simulink model "PVArrayIVTestXaxisShade"  (R2023a)
settings: Solver=VariableStepAuto  StartTime=0.0  StopTime=10.0  RelTol=1e-3
undefined symbols (not defined in the file): Rl
libraries: spsSeriesRLCBranchLib x84, spsPVArrayLib x72, spsCurrentMeasurementLib x12, spsVariableResistorLib x12, spsVoltageMeasurementLib x12, SignalEditorBlockLib x1, sps_lib x1
settings Model: Creator=Akbar  LastModifiedBy=Akbar

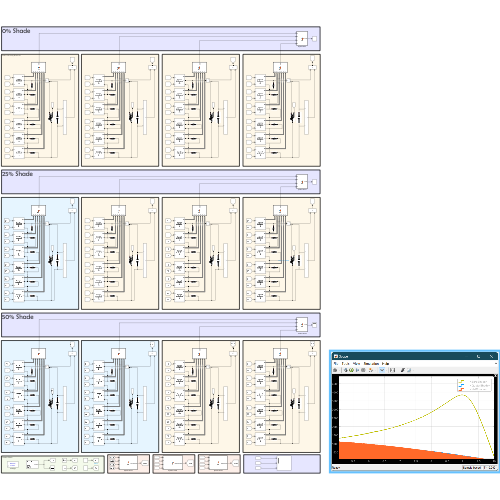
[thumbnail: Simulink's stored preview of the top-level diagram]
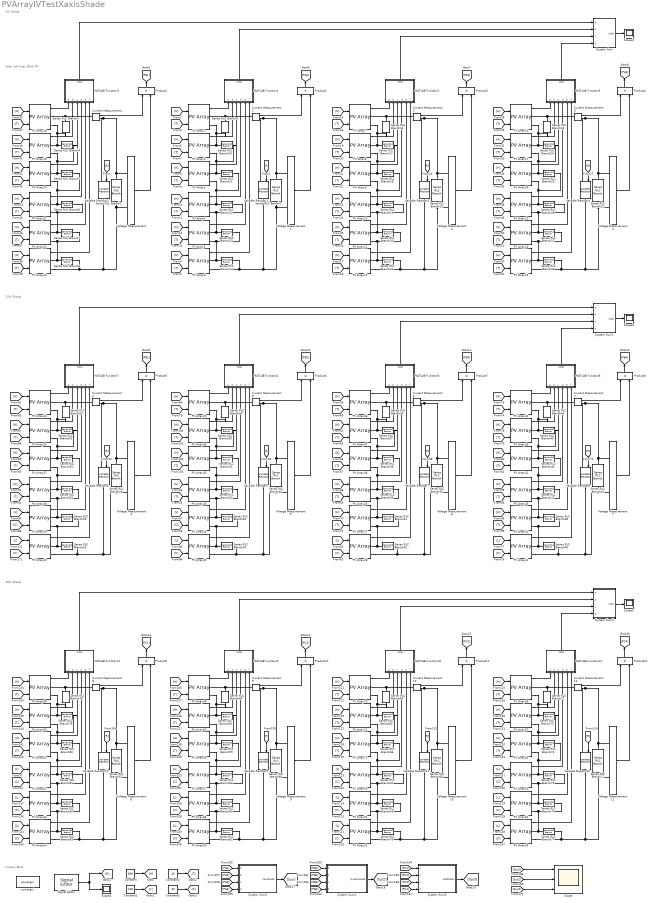
== system PVArrayIVTestXaxisShade ==
  note: Primary Block
  note: 0% Shade
  note: Solar Cell Array Block #1
  note: 25% Shade
  note: 50% Shade
  Constant : Constant  Value=800
  Constant1 : Constant  Value=100
  Constant2 : Constant  Value=45
  Constant3 : Constant  Value=30
  Current Measurement{,1..11} (12 alike) : spsCurrentMeasurementLib/Current Measurement  PhasorSimulation=off  OutputType=Complex  PSBequivalent=0
  MATLAB Function1 : MATLAB Function  TreatAsAtomicUnit=on
  MATLAB Function10 : MATLAB Function  TreatAsAtomicUnit=on
  MATLAB Function11 : MATLAB Function  TreatAsAtomicUnit=on
  MATLAB Function12 : MATLAB Function  TreatAsAtomicUnit=on
  MATLAB Function2 : MATLAB Function  TreatAsAtomicUnit=on
  MATLAB Function3 : MATLAB Function  TreatAsAtomicUnit=on
  MATLAB Function4 : MATLAB Function  TreatAsAtomicUnit=on
  MATLAB Function5 : MATLAB Function  TreatAsAtomicUnit=on
  MATLAB Function6 : MATLAB Function  TreatAsAtomicUnit=on
  MATLAB Function7 : MATLAB Function  TreatAsAtomicUnit=on
  MATLAB Function8 : MATLAB Function  TreatAsAtomicUnit=on
  MATLAB Function9 : MATLAB Function  TreatAsAtomicUnit=on
  PV Array{1..72} (72 alike) : spsPVArrayLib/PV Array  Npar=1  Nser=1  PlotType=array @ 1000 W/m2 & specified temperatures  S_vec="[ 1000  500  100 ]"  Temp_C_vec="[ 45 25  ]"  ModuleName=User-defined  PlotWhenSelected=off  Pm=213.15  Ncell=60  Voc=36.3  Isc=7.84  Vm=29  Im=7.35  beta_Voc_pc=-0.36099  alpha_Isc_pc=0.102  beta_Voc=-0.13104  alpha_Isc=0.0079968  IL=7.8654  I0=2.9273e-10  nI=0.98119  Rsh=313.0553  Rs=0.39381  RobustModel=off  RobustCellTemperature=313.3991  BAL=on  Tc=1e-6  Tfilter=5e-5
  Product{1..12} (12 alike) : Product
  Scope : Scope  NumInputPorts=3
  Scope{2..5} (4 alike) : Scope
  Series RLC Branch{1..2,15,22,29,35,40,43,57,63,68,71} (12 alike) : spsSeriesRLCBranchLib/Series RLC Branch  LConnTagsString=__new0  RConnTagsString=__new0  BranchType=C  Resistance=Rl  Inductance=1e-3  SetiL0=off  InitialCurrent=0  Capacitance=0.01  Setx0=off  InitialVoltage=150  Measurements=Branch voltage and current
  Series RLC Branch{3..14,16..21,23..28,30..34,36..39,41..42,44..56,58..62,64..67,69..70,72..84} (72 alike) : spsSeriesRLCBranchLib/Series RLC Branch  LConnTagsString=__new0  RConnTagsString=__new0  BranchType=C  Resistance=Rl  Inductance=1e-3  SetiL0=off  InitialCurrent=0  Capacitance=1e-2  Setx0=off  InitialVoltage=0  Measurements=Branch voltage and current
  Signal Editor : SignalEditorBlockLib/Signal Editor  FileName=C:\Users\Akbar\Cloud-Drive\School Work\L6 BEng EEE\Semester 1\EEE6016 Renewables\VR\Matlab\SlopeDown1000.mat  ActiveScenario=SlopeHalf  ActiveSignal=Posit  IsBus=off  OutputBusObjectStr=Bus: BusObject  SampleTime=0.0001  ZeroCross=off  OutputAfterFinalValue=Holding final value  Unit=inherit  PreserveSignalName=on  ApplySigPropsToAllScenarios=on
  System Sum : MATLAB Function  TreatAsAtomicUnit=on
  System Sum1 : MATLAB Function  TreatAsAtomicUnit=on
  System Sum2 : MATLAB Function  TreatAsAtomicUnit=on
  System Sum3 : MATLAB Function  TreatAsAtomicUnit=on
  System Sum4 : MATLAB Function  TreatAsAtomicUnit=on
  System Sum5 : MATLAB Function  TreatAsAtomicUnit=on
  Variable Resistor{1..12} (12 alike) : spsVariableResistorLib/Variable Resistor  Rabsmin=1e-3
      settings: LibrarySourceBlock=sps_lib/Passives/Variable Resistor
  Voltage Measurement{,1..11} (12 alike) : spsVoltageMeasurementLib/Voltage Measurement  PhasorSimulation=off  OutputType=Complex  PSBequivalent=0
  powergui : sps_lib/powergui  Priority=1  SimulationMode=Discrete  SampleTime=1e-6  frequency=60  Iterations=50  frequencyindice=0  Pbase=100e6  ErrMax=1e-4  UnitsV=kV  UnitsW=MW  buscounter=0  FunctionMessages=off  echomessages=off  EnableUseOfTLC=off  CurrentSourceSwitches=off  DisableSnubberDevices=off  DisableRonSwitches=off  DisableVfSwitches=off  DisplayEquations=off  AutomaticDiscreteSolvers=off  SolverType=Tustin/Backward Euler (TBE)  Interpol=off  ExternalGateDelay=off  methode=off  Ts=100  x0status=blocks  SPID=on  SwTol=0  HookPort=off  NonlinearTolerance=1e-4  nMaxIteration=100  ContinueOnMaxIteration=off  RestoreLinks=warning  ResistiveCurrentMeasurement=off  Frange=[0:2:500]  Ylog=off  Xlog=on  ShowGrid=off  save=off  variable=ZData  structure=0  ZoomFFT=off  StartTime=0.0  cycles=1  DisplayStyle=1  fundamental=60  FreqAxis=off  MaxFrequency=1000  frequencyindicesteady=1  RmsSteady=1  display=off
  wires:
  PV Array23/1 -> MATLAB Function3/6(f)
  [T] -> PV Array23/2
  [H] -> PV Array18/1
  PV Array19/1 -> MATLAB Function3/2(b)
  PV Array22/1 -> MATLAB Function3/5(e)
  [H] -> PV Array23/1
  [H] -> PV Array21/1
  PV Array20/1 -> MATLAB Function3/3(c)
  [H] -> PV Array22/1
  PV Array21/1 -> MATLAB Function3/4(d)
  [H] -> PV Array20/1
  PV Array18/1 -> MATLAB Function3/1(a)
  [T] -> PV Array19/2
  [H] -> PV Array19/1
  Constant1/1 -> [L]
  Constant/1 -> [H]
  Constant2/1 -> [T]
  Constant3/1 -> [C]
  [T] -> PV Array21/2
  [T] -> PV Array18/2
  [T] -> PV Array20/2
  [T] -> PV Array22/2
  Signal Editor/1 -> [R], Scope2/1
  System Sum/1(total) -> Scope3/1
  [R] -> Variable Resistor2/1
  [R] -> Variable Resistor1/1
  [H] -> PV Array3/1
  PV Array1/1 -> MATLAB Function1/1(a)
  [H] -> PV Array6/1
  [T] -> PV Array1/2
  PV Array4/1 -> MATLAB Function1/4(d)
  [T] -> PV Array4/2
  [T] -> PV Array3/2
  PV Array6/1 -> MATLAB Function1/6(f)
  [T] -> PV Array6/2
  [H] -> PV Array1/1
  [T] -> PV Array5/2
  [H] -> PV Array4/1
  [T] -> PV Array2/2
  PV Array3/1 -> MATLAB Function1/3(c)
  [H] -> PV Array2/1
  PV Array5/1 -> MATLAB Function1/5(e)
  PV Array2/1 -> MATLAB Function1/2(b)
  [H] -> PV Array5/1
  [R] -> Variable Resistor3/1
  [H] -> PV Array9/1
  PV Array7/1 -> MATLAB Function2/1(a)
  [H] -> PV Array12/1
  [T] -> PV Array7/2
  PV Array10/1 -> MATLAB Function2/4(d)
  [T] -> PV Array10/2
  [T] -> PV Array9/2
  PV Array12/1 -> MATLAB Function2/6(f)
  [T] -> PV Array12/2
  [H] -> PV Array7/1
  [T] -> PV Array11/2
  [H] -> PV Array10/1
  [T] -> PV Array8/2
  PV Array9/1 -> MATLAB Function2/3(c)
  [H] -> PV Array8/1
  PV Array11/1 -> MATLAB Function2/5(e)
  PV Array8/1 -> MATLAB Function2/2(b)
  [H] -> PV Array11/1
  [H] -> PV Array17/1
  PV Array24/1 -> MATLAB Function5/3(c)
  [T] -> PV Array17/2
  [H] -> PV Array13/1
  PV Array14/1 -> MATLAB Function5/5(e)
  PV Array15/1 -> MATLAB Function5/6(f)
  [H] -> PV Array15/1
  PV Array16/1 -> MATLAB Function5/1(a)
  [T] -> PV Array14/2
  PV Array13/1 -> MATLAB Function5/4(d)
  [H] -> PV Array16/1
  [R] -> Variable Resistor4/1
  [H] -> PV Array24/1
  [H] -> PV Array14/1
  [T] -> PV Array13/2
  PV Array17/1 -> MATLAB Function5/2(b)
  [T] -> PV Array15/2
  [T] -> PV Array24/2
  [T] -> PV Array16/2
  MATLAB Function5/1(total) -> System Sum/4(d)
  MATLAB Function2/1(total) -> System Sum/3(c)
  MATLAB Function1/1(total) -> System Sum/2(b)
  MATLAB Function3/1(total) -> System Sum/1(a)
  Voltage Measurement/1 -> Product1/2
  Current Measurement/1 -> Product1/1
  Voltage Measurement1/1 -> Product2/2
  Current Measurement1/1 -> Product2/1
  Voltage Measurement2/1 -> Product3/2
  Current Measurement2/1 -> Product3/1
  Voltage Measurement3/1 -> Product4/2
  Current Measurement3/1 -> Product4/1
  [H] -> PV Array29/1
  PV Array30/1 -> MATLAB Function8/5(e)
  PV Array36/1 -> MATLAB Function4/2(b)
  [H] -> PV Array25/1
  [T] -> PV Array43/2
  PV Array45/1 -> MATLAB Function4/6(f)
  PV Array43/1 -> MATLAB Function4/4(d)
  [T] -> PV Array36/2
  [R] -> Variable Resistor5/1
  [H] -> PV Array42/1
  [T] -> PV Array25/2
  PV Array25/1 -> MATLAB Function4/1(a)
  [T] -> PV Array42/2
  [H] -> PV Array43/1
  MATLAB Function6/1(total) -> System Sum1/3(c)
  Current Measurement6/1 -> Product7/1
  Current Measurement5/1 -> Product6/1
  PV Array31/1 -> MATLAB Function8/6(f)
  [T] -> PV Array30/2
  PV Array32/1 -> MATLAB Function8/1(a)
  [H] -> PV Array33/1
  MATLAB Function8/1(total) -> System Sum1/4(d)
  PV Array29/1 -> MATLAB Function8/4(d)
  [H] -> PV Array30/1
  [R] -> Variable Resistor8/1
  [H] -> PV Array41/1
  [T] -> PV Array29/2
  Current Measurement7/1 -> Product8/1
  Voltage Measurement7/1 -> Product8/2
  [T] -> PV Array32/2
  Voltage Measurement5/1 -> Product6/2
  Current Measurement4/1 -> Product5/1
  PV Array34/1 -> MATLAB Function7/1(a)
  PV Array37/1 -> MATLAB Function7/3(c)
  [H] -> PV Array36/1
  PV Array40/1 -> MATLAB Function7/6(f)
  Voltage Measurement6/1 -> Product7/2
  PV Array42/1 -> MATLAB Function4/3(c)
  PV Array39/1 -> MATLAB Function7/5(e)
  PV Array35/1 -> MATLAB Function7/2(b)
  MATLAB Function7/1(total) -> System Sum1/1(a)
  Voltage Measurement4/1 -> Product5/2
  [T] -> PV Array33/2
  [H] -> PV Array47/1
  PV Array48/1 -> MATLAB Function6/3(c)
  [T] -> PV Array47/2
  [H] -> PV Array26/1
  PV Array27/1 -> MATLAB Function6/5(e)
  [H] -> PV Array32/1
  PV Array28/1 -> MATLAB Function6/6(f)
  [T] -> PV Array27/2
  [H] -> PV Array46/1
  [H] -> PV Array48/1
  [R] -> Variable Resistor7/1
  [R] -> Variable Resistor6/1
  [H] -> PV Array27/1
  PV Array38/1 -> MATLAB Function7/4(d)
  PV Array47/1 -> MATLAB Function6/2(b)
  [T] -> PV Array48/2
  [T] -> PV Array46/2
  [T] -> PV Array26/2
  PV Array44/1 -> MATLAB Function4/5(e)
  PV Array26/1 -> MATLAB Function6/4(d)
  PV Array33/1 -> MATLAB Function8/2(b)
  PV Array41/1 -> MATLAB Function8/3(c)
  MATLAB Function4/1(total) -> System Sum1/2(b)
  PV Array46/1 -> MATLAB Function6/1(a)
  System Sum1/1(total) -> Scope4/1
  [T] -> PV Array41/2
  PV Array54/1 -> MATLAB Function12/5(e)
  PV Array60/1 -> MATLAB Function9/2(b)
  PV Array69/1 -> MATLAB Function9/6(f)
  PV Array67/1 -> MATLAB Function9/4(d)
  [R] -> Variable Resistor9/1
  PV Array49/1 -> MATLAB Function9/1(a)
  MATLAB Function10/1(total) -> System Sum2/3(c)
  Current Measurement10/1 -> Product11/1
  Current Measurement9/1 -> Product10/1
  PV Array55/1 -> MATLAB Function12/6(f)
  PV Array56/1 -> MATLAB Function12/1(a)
  [H] -> PV Array57/1
  MATLAB Function12/1(total) -> System Sum2/4(d)
  PV Array53/1 -> MATLAB Function12/4(d)
  [R] -> Variable Resistor12/1
  Current Measurement11/1 -> Product12/1
  Voltage Measurement11/1 -> Product12/2
  [T] -> PV Array56/2
  Voltage Measurement9/1 -> Product10/2
  Current Measurement8/1 -> Product9/1
  PV Array58/1 -> MATLAB Function11/1(a)
  PV Array61/1 -> MATLAB Function11/3(c)
  PV Array64/1 -> MATLAB Function11/6(f)
  Voltage Measurement10/1 -> Product11/2
  PV Array66/1 -> MATLAB Function9/3(c)
  PV Array63/1 -> MATLAB Function11/5(e)
  PV Array59/1 -> MATLAB Function11/2(b)
  MATLAB Function11/1(total) -> System Sum2/1(a)
  Voltage Measurement8/1 -> Product9/2
  [T] -> PV Array57/2
  [H] -> PV Array71/1
  PV Array72/1 -> MATLAB Function10/3(c)
  [T] -> PV Array71/2
  PV Array51/1 -> MATLAB Function10/5(e)
  [H] -> PV Array56/1
  PV Array52/1 -> MATLAB Function10/6(f)
  [H] -> PV Array70/1
  [R] -> Variable Resistor11/1
  [R] -> Variable Resistor10/1
  PV Array62/1 -> MATLAB Function11/4(d)
  PV Array71/1 -> MATLAB Function10/2(b)
  [T] -> PV Array70/2
  PV Array68/1 -> MATLAB Function9/5(e)
  PV Array50/1 -> MATLAB Function10/4(d)
  PV Array57/1 -> MATLAB Function12/2(b)
  PV Array65/1 -> MATLAB Function12/3(c)
  MATLAB Function9/1(total) -> System Sum2/2(b)
  PV Array70/1 -> MATLAB Function10/1(a)
  System Sum2/1(total) -> Scope5/1
  Product1/1 -> [PA1]
  Product2/1 -> [PA2]
  Product3/1 -> [PA3]
  Product4/1 -> [PA4]
  Product5/1 -> [PB1]
  Product6/1 -> [PB2]
  Product7/1 -> [PB3]
  Product8/1 -> [PB4]
  Product9/1 -> [PC1]
  Product10/1 -> [PC2]
  Product11/1 -> [PC3]
  Product12/1 -> [PC4]
  [PA1] -> System Sum3/1(a)
  [PA2] -> System Sum3/2(b)
  [PA3] -> System Sum3/3(c)
  [PA4] -> System Sum3/4(d)
  System Sum3/1(ZeroShade) -> [Sys1]
  [PB3] -> System Sum4/3(c)
  [PB1] -> System Sum4/1(a)
  [PB4] -> System Sum4/4(d)
  System Sum4/1(QuaterShade) -> [Sys2]
  [PB2] -> System Sum4/2(b)
  System Sum5/1(HalfShade) -> [Sys3]
  [PC2] -> System Sum5/2(b)
  [PC1] -> System Sum5/1(a)
  [PC4] -> System Sum5/4(d)
  [PC3] -> System Sum5/3(c)
  [Sys1] -> Scope/1
  [Sys2] -> Scope/2
  [Sys3] -> Scope/3
  [H] -> PV Array37/1
  [T] -> PV Array35/2
  [T] -> PV Array37/2
  [L] -> PV Array40/1
  [T] -> PV Array38/2
  [H] -> PV Array35/1
  [H] -> PV Array34/1
  [H] -> PV Array38/1
  [C] -> PV Array40/2
  [T] -> PV Array34/2
  [H] -> PV Array61/1
  [T] -> PV Array59/2
  [T] -> PV Array61/2
  [H] -> PV Array59/1
  [H] -> PV Array58/1
  [T] -> PV Array58/2
  [T] -> PV Array60/2
  [H] -> PV Array60/1
  [H] -> PV Array49/1
  [T] -> PV Array49/2
  [L] -> PV Array45/1
  [C] -> PV Array45/2
  [L] -> PV Array28/1
  [C] -> PV Array28/2
  [L] -> PV Array31/1
  [C] -> PV Array31/2
  [L] -> PV Array39/1
  [C] -> PV Array39/2
  [L] -> PV Array44/1
  [C] -> PV Array44/2
  [L] -> PV Array62/1
  [C] -> PV Array62/2
  [L] -> PV Array63/1
  [C] -> PV Array63/2
  [L] -> PV Array64/1
  [C] -> PV Array64/2
  [L] -> PV Array69/1
  [C] -> PV Array67/2
  [H] -> PV Array66/1
  [C] -> PV Array68/2
  [T] -> PV Array66/2
  [L] -> PV Array67/1
  [L] -> PV Array68/1
  [C] -> PV Array69/2
  [L] -> PV Array52/1
  [C] -> PV Array50/2
  [H] -> PV Array72/1
  [C] -> PV Array51/2
  [T] -> PV Array72/2
  [L] -> PV Array50/1
  [L] -> PV Array51/1
  [C] -> PV Array52/2
  [L] -> PV Array55/1
  [C] -> PV Array53/2
  [H] -> PV Array65/1
  [C] -> PV Array54/2
  [T] -> PV Array65/2
  [L] -> PV Array53/1
  [L] -> PV Array54/1
  [C] -> PV Array55/2
  connections:
  Series RLC Branch1/RConn1 -- Voltage Measurement/LConn2 -- Series RLC Branch8/RConn1 -- PV Array23/RConn2 -- Variable Resistor2/RConn1
  Current Measurement/RConn1 -- Variable Resistor2/LConn1 -- Voltage Measurement/LConn1 -- Series RLC Branch1/LConn1
  PV Array20/RConn2 -- Series RLC Branch5/RConn1 -- Series RLC Branch6/LConn1 -- PV Array21/RConn1
  PV Array22/RConn1 -- Series RLC Branch7/LConn1 -- Series RLC Branch6/RConn1 -- PV Array21/RConn2
  PV Array18/RConn2 -- Series RLC Branch3/RConn1 -- Series RLC Branch4/LConn1 -- PV Array19/RConn1
  PV Array19/RConn2 -- Series RLC Branch4/RConn1 -- Series RLC Branch5/LConn1 -- PV Array20/RConn1
  PV Array22/RConn2 -- Series RLC Branch7/RConn1 -- Series RLC Branch8/LConn1 -- PV Array23/RConn1
  Current Measurement/LConn1 -- Series RLC Branch3/LConn1 -- PV Array18/RConn1
  PV Array3/RConn1 -- Series RLC Branch10/RConn1 -- PV Array2/RConn2 -- Series RLC Branch11/LConn1
  PV Array6/RConn1 -- Series RLC Branch14/LConn1 -- PV Array5/RConn2 -- Series RLC Branch13/RConn1
  PV Array2/RConn1 -- Series RLC Branch9/RConn1 -- PV Array1/RConn2 -- Series RLC Branch10/LConn1
  PV Array4/RConn2 -- Series RLC Branch13/LConn1 -- PV Array5/RConn1 -- Series RLC Branch12/RConn1
  PV Array4/RConn1 -- Series RLC Branch11/RConn1 -- PV Array3/RConn2 -- Series RLC Branch12/LConn1
  PV Array1/RConn1 -- Series RLC Branch9/LConn1 -- Current Measurement1/LConn1
  Variable Resistor1/RConn1 -- Series RLC Branch14/RConn1 -- PV Array6/RConn2 -- Voltage Measurement1/LConn2 -- Series RLC Branch2/RConn1
  Series RLC Branch2/LConn1 -- Voltage Measurement1/LConn1 -- Variable Resistor1/LConn1 -- Current Measurement1/RConn1
  PV Array9/RConn1 -- Series RLC Branch17/RConn1 -- PV Array8/RConn2 -- Series RLC Branch18/LConn1
  PV Array12/RConn1 -- Series RLC Branch21/LConn1 -- PV Array11/RConn2 -- Series RLC Branch20/RConn1
  PV Array8/RConn1 -- Series RLC Branch16/RConn1 -- PV Array7/RConn2 -- Series RLC Branch17/LConn1
  PV Array10/RConn2 -- Series RLC Branch20/LConn1 -- PV Array11/RConn1 -- Series RLC Branch19/RConn1
  PV Array10/RConn1 -- Series RLC Branch18/RConn1 -- PV Array9/RConn2 -- Series RLC Branch19/LConn1
  PV Array7/RConn1 -- Series RLC Branch16/LConn1 -- Current Measurement2/LConn1
  Variable Resistor3/RConn1 -- Series RLC Branch21/RConn1 -- PV Array12/RConn2 -- Voltage Measurement2/LConn2 -- Series RLC Branch15/RConn1
  Series RLC Branch15/LConn1 -- Voltage Measurement2/LConn1 -- Variable Resistor3/LConn1 -- Current Measurement2/RConn1
  PV Array24/RConn1 -- Series RLC Branch25/LConn1 -- Series RLC Branch24/RConn1 -- PV Array17/RConn2
  PV Array17/RConn1 -- Series RLC Branch24/LConn1 -- Series RLC Branch23/RConn1 -- PV Array16/RConn2
  PV Array15/RConn1 -- Series RLC Branch28/LConn1 -- PV Array14/RConn2 -- Series RLC Branch27/RConn1
  Series RLC Branch22/RConn1 -- Voltage Measurement3/LConn2 -- Variable Resistor4/RConn1 -- Series RLC Branch28/RConn1 -- PV Array15/RConn2
  Series RLC Branch22/LConn1 -- Voltage Measurement3/LConn1 -- Variable Resistor4/LConn1 -- Current Measurement3/RConn1
  PV Array13/RConn1 -- Series RLC Branch26/LConn1 -- Series RLC Branch25/RConn1 -- PV Array24/RConn2
  PV Array16/RConn1 -- Series RLC Branch23/LConn1 -- Current Measurement3/LConn1
  PV Array13/RConn2 -- Series RLC Branch26/RConn1 -- Series RLC Branch27/LConn1 -- PV Array14/RConn1
  Series RLC Branch40/RConn1 -- Voltage Measurement5/LConn2 -- Series RLC Branch34/RConn1 -- PV Array45/RConn2 -- Variable Resistor5/RConn1
  PV Array33/RConn1 -- Series RLC Branch45/LConn1 -- Series RLC Branch44/RConn1 -- PV Array32/RConn2
  PV Array43/RConn1 -- Series RLC Branch32/LConn1 -- Series RLC Branch31/RConn1 -- PV Array42/RConn2
  Series RLC Branch43/LConn1 -- Voltage Measurement7/LConn1 -- Variable Resistor8/LConn1 -- Current Measurement7/RConn1
  PV Array41/RConn1 -- Series RLC Branch46/LConn1 -- Series RLC Branch45/RConn1 -- PV Array33/RConn2
  PV Array32/RConn1 -- Series RLC Branch44/LConn1 -- Current Measurement7/LConn1
  Series RLC Branch40/LConn1 -- Voltage Measurement5/LConn1 -- Variable Resistor5/LConn1 -- Current Measurement5/RConn1
  PV Array45/RConn1 -- Series RLC Branch34/LConn1 -- PV Array44/RConn2 -- Series RLC Branch33/RConn1
  PV Array35/RConn1 -- Series RLC Branch50/RConn1 -- PV Array34/RConn2 -- Series RLC Branch51/LConn1
  PV Array30/RConn1 -- Series RLC Branch48/LConn1 -- Series RLC Branch47/RConn1 -- PV Array29/RConn2
  PV Array36/RConn1 -- Series RLC Branch56/RConn1 -- PV Array25/RConn2 -- Series RLC Branch30/LConn1
  PV Array38/RConn1 -- Series RLC Branch53/LConn1 -- Series RLC Branch52/RConn1 -- PV Array37/RConn2
  Series RLC Branch29/LConn1 -- Variable Resistor6/LConn1 -- Current Measurement4/RConn1 -- Voltage Measurement4/LConn1
  Variable Resistor6/RConn1 -- Series RLC Branch55/RConn1 -- PV Array40/RConn2 -- Voltage Measurement4/LConn2 -- Series RLC Branch29/RConn1
  PV Array47/RConn1 -- Series RLC Branch37/LConn1 -- Series RLC Branch36/RConn1 -- PV Array46/RConn2
  PV Array37/RConn1 -- Series RLC Branch51/RConn1 -- PV Array35/RConn2 -- Series RLC Branch52/LConn1
  PV Array42/RConn1 -- Series RLC Branch30/RConn1 -- PV Array36/RConn2 -- Series RLC Branch31/LConn1
  Series RLC Branch35/LConn1 -- Voltage Measurement6/LConn1 -- Variable Resistor7/LConn1 -- Current Measurement6/RConn1
  PV Array43/RConn2 -- Series RLC Branch33/LConn1 -- PV Array44/RConn1 -- Series RLC Branch32/RConn1
  PV Array34/RConn1 -- Series RLC Branch50/LConn1 -- Current Measurement4/LConn1
  PV Array26/RConn2 -- Series RLC Branch41/LConn1 -- PV Array27/RConn1 -- Series RLC Branch39/RConn1
  PV Array26/RConn1 -- Series RLC Branch38/RConn1 -- PV Array48/RConn2 -- Series RLC Branch39/LConn1
  Series RLC Branch35/RConn1 -- Voltage Measurement6/LConn2 -- Series RLC Branch42/RConn1 -- PV Array28/RConn2 -- Variable Resistor7/RConn1
  PV Array38/RConn2 -- Series RLC Branch53/RConn1 -- Series RLC Branch54/LConn1 -- PV Array39/RConn1
  PV Array31/RConn1 -- Series RLC Branch49/LConn1 -- PV Array30/RConn2 -- Series RLC Branch48/RConn1
  PV Array28/RConn1 -- Series RLC Branch42/LConn1 -- PV Array27/RConn2 -- Series RLC Branch41/RConn1
  PV Array40/RConn1 -- Series RLC Branch55/LConn1 -- PV Array39/RConn2 -- Series RLC Branch54/RConn1
  PV Array25/RConn1 -- Series RLC Branch56/LConn1 -- Current Measurement5/LConn1
  PV Array48/RConn1 -- Series RLC Branch37/RConn1 -- PV Array47/RConn2 -- Series RLC Branch38/LConn1
  PV Array29/RConn1 -- Series RLC Branch47/LConn1 -- Series RLC Branch46/RConn1 -- PV Array41/RConn2
  PV Array31/RConn2 -- Variable Resistor8/RConn1 -- Voltage Measurement7/LConn2 -- Series RLC Branch43/RConn1 -- Series RLC Branch49/RConn1
  PV Array46/RConn1 -- Series RLC Branch36/LConn1 -- Current Measurement6/LConn1
  Series RLC Branch68/RConn1 -- Voltage Measurement9/LConn2 -- Variable Resistor9/RConn1 -- Series RLC Branch62/RConn1 -- PV Array69/RConn2
  PV Array57/RConn1 -- Series RLC Branch73/LConn1 -- Series RLC Branch72/RConn1 -- PV Array56/RConn2
  PV Array67/RConn1 -- Series RLC Branch60/LConn1 -- Series RLC Branch59/RConn1 -- PV Array66/RConn2
  Series RLC Branch71/LConn1 -- Voltage Measurement11/LConn1 -- Variable Resistor12/LConn1 -- Current Measurement11/RConn1
  PV Array65/RConn1 -- Series RLC Branch74/LConn1 -- Series RLC Branch73/RConn1 -- PV Array57/RConn2
  PV Array56/RConn1 -- Series RLC Branch72/LConn1 -- Current Measurement11/LConn1
  Series RLC Branch68/LConn1 -- Voltage Measurement9/LConn1 -- Variable Resistor9/LConn1 -- Current Measurement9/RConn1
  PV Array69/RConn1 -- Series RLC Branch62/LConn1 -- PV Array68/RConn2 -- Series RLC Branch61/RConn1
  PV Array59/RConn1 -- Series RLC Branch78/RConn1 -- PV Array58/RConn2 -- Series RLC Branch79/LConn1
  PV Array54/RConn1 -- Series RLC Branch76/LConn1 -- Series RLC Branch75/RConn1 -- PV Array53/RConn2
  PV Array60/RConn1 -- Series RLC Branch84/RConn1 -- PV Array49/RConn2 -- Series RLC Branch58/LConn1
  PV Array62/RConn1 -- Series RLC Branch81/LConn1 -- Series RLC Branch80/RConn1 -- PV Array61/RConn2
  Series RLC Branch57/LConn1 -- Variable Resistor10/LConn1 -- Current Measurement8/RConn1 -- Voltage Measurement8/LConn1
  Variable Resistor10/RConn1 -- Series RLC Branch83/RConn1 -- PV Array64/RConn2 -- Voltage Measurement8/LConn2 -- Series RLC Branch57/RConn1
  PV Array71/RConn1 -- Series RLC Branch65/LConn1 -- Series RLC Branch64/RConn1 -- PV Array70/RConn2
  PV Array61/RConn1 -- Series RLC Branch79/RConn1 -- PV Array59/RConn2 -- Series RLC Branch80/LConn1
  PV Array66/RConn1 -- Series RLC Branch58/RConn1 -- PV Array60/RConn2 -- Series RLC Branch59/LConn1
  Series RLC Branch63/LConn1 -- Voltage Measurement10/LConn1 -- Variable Resistor11/LConn1 -- Current Measurement10/RConn1
  PV Array67/RConn2 -- Series RLC Branch61/LConn1 -- PV Array68/RConn1 -- Series RLC Branch60/RConn1
  PV Array58/RConn1 -- Series RLC Branch78/LConn1 -- Current Measurement8/LConn1
  PV Array50/RConn2 -- Series RLC Branch69/LConn1 -- PV Array51/RConn1 -- Series RLC Branch67/RConn1
  PV Array50/RConn1 -- Series RLC Branch66/RConn1 -- PV Array72/RConn2 -- Series RLC Branch67/LConn1
  Series RLC Branch63/RConn1 -- Voltage Measurement10/LConn2 -- Series RLC Branch70/RConn1 -- PV Array52/RConn2 -- Variable Resistor11/RConn1
  PV Array62/RConn2 -- Series RLC Branch81/RConn1 -- Series RLC Branch82/LConn1 -- PV Array63/RConn1
  PV Array55/RConn1 -- Series RLC Branch77/LConn1 -- PV Array54/RConn2 -- Series RLC Branch76/RConn1
  PV Array52/RConn1 -- Series RLC Branch70/LConn1 -- PV Array51/RConn2 -- Series RLC Branch69/RConn1
  PV Array64/RConn1 -- Series RLC Branch83/LConn1 -- PV Array63/RConn2 -- Series RLC Branch82/RConn1
  PV Array49/RConn1 -- Series RLC Branch84/LConn1 -- Current Measurement9/LConn1
  PV Array72/RConn1 -- Series RLC Branch65/RConn1 -- PV Array71/RConn2 -- Series RLC Branch66/LConn1
  PV Array53/RConn1 -- Series RLC Branch75/LConn1 -- Series RLC Branch74/RConn1 -- PV Array65/RConn2
  PV Array55/RConn2 -- Series RLC Branch77/RConn1 -- Variable Resistor12/RConn1 -- Voltage Measurement11/LConn2 -- Series RLC Branch71/RConn1
  PV Array70/RConn1 -- Series RLC Branch64/LConn1 -- Current Measurement10/LConn1

== matlab function PVArrayIVTestXaxisShade/MATLAB Function8 ==
  data: a input; total output; b input; c input; d input; e input; f input
function total = fcn(a,b,c,d,e,f)

total = a+b+c+d+e+f;

== matlab function PVArrayIVTestXaxisShade/System Sum1 ==
  data: a input; total output; b input; c input; d input
function total = fcn(a,b,c,d)

total = a+b+c+d;

== matlab function PVArrayIVTestXaxisShade/MATLAB Function1 ==
  data: a input; total output; b input; c input; d input; e input; f input
function total = fcn(a,b,c,d,e,f)

total = a+b+c+d+e+f;

== matlab function PVArrayIVTestXaxisShade/MATLAB Function10 ==
  data: a input; total output; b input; c input; d input; e input; f input
function total = fcn(a,b,c,d,e,f)

total = a+b+c+d+e+f;

== matlab function PVArrayIVTestXaxisShade/MATLAB Function11 ==
  data: a input; total output; b input; c input; d input; e input; f input
function total = fcn(a,b,c,d,e,f)

total = a+b+c+d+e+f;

== matlab function PVArrayIVTestXaxisShade/MATLAB Function12 ==
  data: a input; total output; b input; c input; d input; e input; f input
function total = fcn(a,b,c,d,e,f)

total = a+b+c+d+e+f;

== matlab function PVArrayIVTestXaxisShade/MATLAB Function9 ==
  data: a input; total output; b input; c input; d input; e input; f input
function total = fcn(a,b,c,d,e,f)

total = a+b+c+d+e+f;

== matlab function PVArrayIVTestXaxisShade/System Sum2 ==
  data: a input; total output; b input; c input; d input
function total = fcn(a,b,c,d)

total = a+b+c+d;

== matlab function PVArrayIVTestXaxisShade/System Sum3 ==
  data: a input; ZeroShade output; b input; c input; d input
function ZeroShade = fcn(a,b,c,d)

ZeroShade = a+b+c+d;

== matlab function PVArrayIVTestXaxisShade/System Sum4 ==
  data: a input; QuaterShade output; b input; c input; d input
function QuaterShade = fcn(a,b,c,d)

QuaterShade = a+b+c+d;

== matlab function PVArrayIVTestXaxisShade/System Sum5 ==
  data: a input; HalfShade output; b input; c input; d input
function HalfShade = fcn(a,b,c,d)

HalfShade = a+b+c+d;

== matlab function PVArrayIVTestXaxisShade/MATLAB Function2 ==
  data: a input; total output; b input; c input; d input; e input; f input
function total = fcn(a,b,c,d,e,f)

total = a+b+c+d+e+f;

== matlab function PVArrayIVTestXaxisShade/MATLAB Function5 ==
  data: a input; total output; b input; c input; d input; e input; f input
function total = fcn(a,b,c,d,e,f)

total = a+b+c+d+e+f;

== matlab function PVArrayIVTestXaxisShade/MATLAB Function3 ==
  data: a input; total output; b input; c input; d input; e input; f input
function total = fcn(a,b,c,d,e,f)

total = a+b+c+d+e+f;

== matlab function PVArrayIVTestXaxisShade/System Sum ==
  data: a input; total output; b input; c input; d input
function total = fcn(a,b,c,d)

total = a+b+c+d;

== matlab function PVArrayIVTestXaxisShade/MATLAB Function4 ==
  data: a input; total output; b input; c input; d input; e input; f input
function total = fcn(a,b,c,d,e,f)

total = a+b+c+d+e+f;

== matlab function PVArrayIVTestXaxisShade/MATLAB Function6 ==
  data: a input; total output; b input; c input; d input; e input; f input
function total = fcn(a,b,c,d,e,f)

total = a+b+c+d+e+f;

== matlab function PVArrayIVTestXaxisShade/MATLAB Function7 ==
  data: a input; total output; b input; c input; d input; e input; f input
function total = fcn(a,b,c,d,e,f)

total = a+b+c+d+e+f;
